simulink model "dsp_channelized_receiver_"  (R2021a)
settings: Solver=VariableStepAuto  StartTime=0.0  StopTime=sim_time  RelTol=1e-3
values from neighbouring files (symbols this model uses):
  sim_time = 1e-3    (= 0.001)    [rx_dsp_core_init_hw.m]
  ts = 1/fs    (= 2.5e-10)    [rx_dsp_core_init_hw.m]
undefined symbols (not defined in the file or in its folder): es1
libraries: xbsIndex_r4 x267, dspsrcs4 x3, simulink x1, dspswit3 x1
(part 1 of 2)
settings Model: ModifiedByFormat=HosseinBehshti  Creator=HosseinBehshti  LastModifiedBy=HosseinBehshti

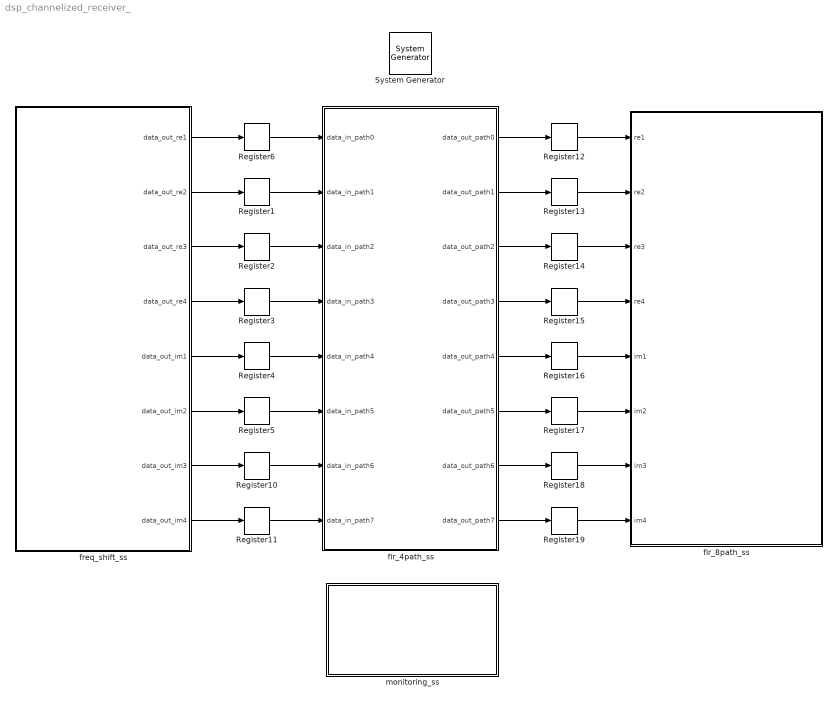
== system dsp_channelized_receiver_ ==
  " System Generator" : xbsIndex_r4/ System Generator  Tag=genX  xilinxfamily=zynquplusRFSOCes1  part=xczu48dr  speed=-2-e-es1  package=fsvg1517  synthesis_tool=Vivado  clock_wrapper=Clock Enables  directory=./netlist  proj_type=Vivado  Synth_file=Vivado Synthesis Defaults  Impl_file=Vivado Implementation Defaults  testbench=off  simulink_period=ts  sysclk_period=2  dcm_input_clock_period=10  incr_netlist=off  trim_vbits=Everywhere in SubSystem  dbl_ovrd=According to Block Masks  core_generation=According to Block Masks  run_coregen=off  deprecated_control=off  eval_field=0  block_type=sysgen
  Register{1..6,10..19} (16 alike) : xbsIndex_r4/Register  init=0  rst=off  en=off  dbl_ovrd=off  block_type=register
  fir_4path_ss : Subsystem
  fir_8path_ss : Subsystem
  freq_shift_ss : Subsystem
  monitoring_ss : Subsystem
  wires:
  Register6/1 -> fir_4path_ss/1(data_in_path0)
  Register1/1 -> fir_4path_ss/2(data_in_path1)
  Register2/1 -> fir_4path_ss/3(data_in_path2)
  Register3/1 -> fir_4path_ss/4(data_in_path3)
  Register4/1 -> fir_4path_ss/5(data_in_path4)
  Register5/1 -> fir_4path_ss/6(data_in_path5)
  Register10/1 -> fir_4path_ss/7(data_in_path6)
  Register11/1 -> fir_4path_ss/8(data_in_path7)
  fir_4path_ss/1(data_out_path0) -> Register12/1
  fir_4path_ss/2(data_out_path1) -> Register13/1
  fir_4path_ss/3(data_out_path2) -> Register14/1
  fir_4path_ss/4(data_out_path3) -> Register15/1
  fir_4path_ss/5(data_out_path4) -> Register16/1
  fir_4path_ss/6(data_out_path5) -> Register17/1
  fir_4path_ss/7(data_out_path6) -> Register18/1
  fir_4path_ss/8(data_out_path7) -> Register19/1
  Register12/1 -> fir_8path_ss/1(re1)
  Register13/1 -> fir_8path_ss/2(re2)
  Register14/1 -> fir_8path_ss/3(re3)
  Register17/1 -> fir_8path_ss/6(im2)
  Register16/1 -> fir_8path_ss/5(im1)
  Register15/1 -> fir_8path_ss/4(re4)
  Register19/1 -> fir_8path_ss/8(im4)
  Register18/1 -> fir_8path_ss/7(im3)
  freq_shift_ss/1(data_out_re1) -> Register6/1
  freq_shift_ss/2(data_out_re2) -> Register1/1
  freq_shift_ss/3(data_out_re3) -> Register2/1
  freq_shift_ss/4(data_out_re4) -> Register3/1
  freq_shift_ss/5(data_out_im1) -> Register4/1
  freq_shift_ss/6(data_out_im2) -> Register5/1
  freq_shift_ss/7(data_out_im3) -> Register10/1
  freq_shift_ss/8(data_out_im4) -> Register11/1

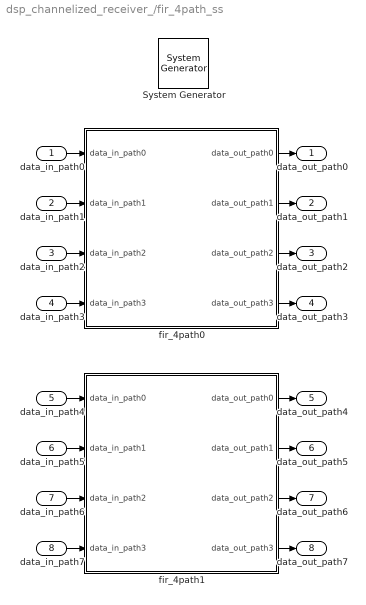
== system dsp_channelized_receiver_/fir_4path_ss ==
  data_in_path0 : Inport
  data_in_path1 : Inport  Port=2
  data_in_path2 : Inport  Port=3
  data_in_path3 : Inport  Port=4
  data_in_path4 : Inport  Port=5
  data_in_path5 : Inport  Port=6
  data_in_path6 : Inport  Port=7
  data_in_path7 : Inport  Port=8
  " System Generator" : xbsIndex_r4/ System Generator  Tag=genX  xilinxfamily=zynquplusRFSOCes1  part=xczu48dr  speed=-2-e-es1  package=fsvg1517  synthesis_tool=Vivado  clock_wrapper=Clock Enables  directory=./netlist  proj_type=Vivado  Synth_file=Vivado Synthesis Defaults  Impl_file=Vivado Implementation Defaults  testbench=off  simulink_period=ts*4  sysclk_period=2*4  dcm_input_clock_period=10  incr_netlist=off  trim_vbits=Everywhere in SubSystem  dbl_ovrd=According to Block Masks  core_generation=According to Block Masks  run_coregen=off  deprecated_control=off  eval_field=0  block_type=sysgen
  fir_4path0 : Subsystem
  fir_4path1 : Subsystem
  data_out_path0 : Outport
  data_out_path1 : Outport  Port=2
  data_out_path2 : Outport  Port=3
  data_out_path3 : Outport  Port=4
  data_out_path4 : Outport  Port=5
  data_out_path5 : Outport  Port=6
  data_out_path6 : Outport  Port=7
  data_out_path7 : Outport  Port=8
  wires:
  data_in_path3/1 -> fir_4path0/4(data_in_path3)
  data_in_path7/1 -> fir_4path1/4(data_in_path3)
  data_in_path4/1 -> fir_4path1/1(data_in_path0)
  fir_4path1/3(data_out_path2) -> data_out_path6/1
  fir_4path1/2(data_out_path1) -> data_out_path5/1
  data_in_path5/1 -> fir_4path1/2(data_in_path1)
  data_in_path6/1 -> fir_4path1/3(data_in_path2)
  fir_4path1/4(data_out_path3) -> data_out_path7/1
  fir_4path1/1(data_out_path0) -> data_out_path4/1
  data_in_path1/1 -> fir_4path0/2(data_in_path1)
  fir_4path0/1(data_out_path0) -> data_out_path0/1
  data_in_path2/1 -> fir_4path0/3(data_in_path2)
  fir_4path0/3(data_out_path2) -> data_out_path2/1
  data_in_path0/1 -> fir_4path0/1(data_in_path0)
  fir_4path0/2(data_out_path1) -> data_out_path1/1
  fir_4path0/4(data_out_path3) -> data_out_path3/1

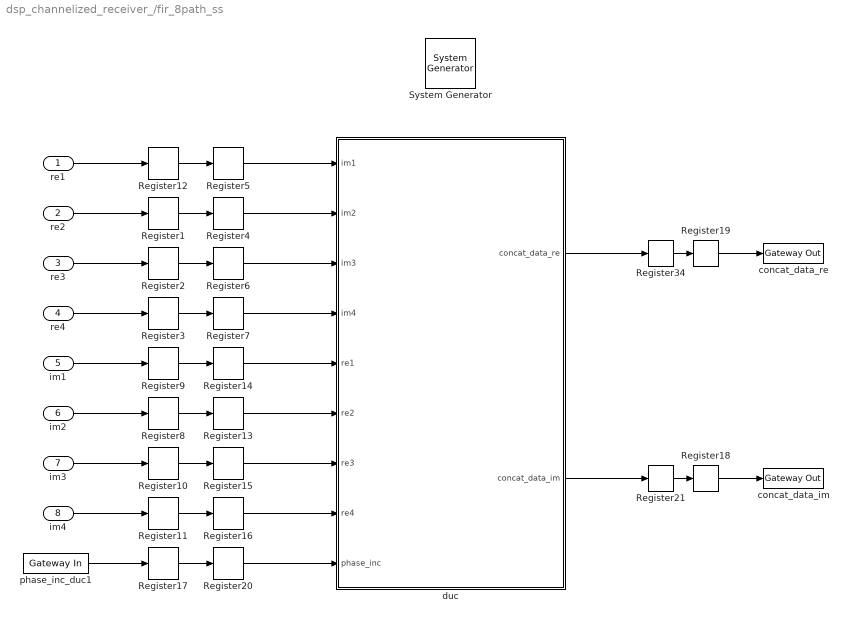
== system dsp_channelized_receiver_/fir_8path_ss ==
  re1 : Inport
  re2 : Inport  Port=2
  re3 : Inport  Port=3
  re4 : Inport  Port=4
  im1 : Inport  Port=5
  im2 : Inport  Port=6
  im3 : Inport  Port=7
  im4 : Inport  Port=8
  " System Generator" : xbsIndex_r4/ System Generator  Tag=genX  xilinxfamily=zynquplusRFSOCes1  part=xczu48dr  speed=-2-e-es1  package=fsvg1517  synthesis_tool=Vivado  clock_wrapper=Clock Enables  directory=./netlist  proj_type=Vivado  Synth_file=Vivado Synthesis Defaults  Impl_file=Vivado Implementation Defaults  testbench=off  simulink_period=ts  sysclk_period=2  dcm_input_clock_period=10  incr_netlist=off  trim_vbits=Everywhere in SubSystem  dbl_ovrd=According to Block Masks  core_generation=According to Block Masks  run_coregen=off  deprecated_control=off  eval_field=0  block_type=sysgen
  Register{1..21,34} (22 alike) : xbsIndex_r4/Register  init=0  rst=off  en=off  dbl_ovrd=off  block_type=register
  concat_data_im : xbsIndex_r4/Gateway Out  inherit_from_input=off  hdl_port=on  rows=1  columns=1  UseAsDAC=off  DACChannel='1'  interface=None  automatic_assignment=on  address_offset=hex2dec('00')  intf_name=''  intf_description=''  timing_constraint=None  locs_specified=off  LOCs={}  io_standard={}  block_type=gatewayout
  concat_data_re : xbsIndex_r4/Gateway Out  inherit_from_input=off  hdl_port=on  rows=1  columns=1  UseAsDAC=off  DACChannel='1'  interface=None  automatic_assignment=on  address_offset=hex2dec('00')  intf_name=''  intf_description=''  timing_constraint=None  locs_specified=off  LOCs={}  io_standard={}  block_type=gatewayout
  duc : Subsystem
  phase_inc_duc1 : xbsIndex_r4/Gateway In  gui_display_data_type=Fixed-point  arith_type=Unsigned  n_bits=ddc_phase_width  bin_pt=ddc_phase_width  preci_type=Single  exp_width=8  frac_width=24  rows=1  columns=1  quantization="Round  (unbiased: +/- Inf)"  overflow=Saturate  period=ts  UseAsADC=off  ADCChannel='1'  interface=None  automatic_assignment=on  address_offset=hex2dec('00')  intf_name=''  intf_description=''  default_value=0  timing_constraint=None  locs_specified=off  LOCs={}  io_standard={}  inherit_from_input=off  hdl_port=on  dbl_ovrd=off  block_type=gatewayin
  wires:
  re1/1 -> Register12/1
  re3/1 -> Register2/1
  re2/1 -> Register1/1
  re4/1 -> Register3/1
  Register12/1 -> Register5/1
  Register1/1 -> Register4/1
  Register2/1 -> Register6/1
  Register3/1 -> Register7/1
  Register11/1 -> Register16/1
  Register10/1 -> Register15/1
  Register8/1 -> Register13/1
  Register9/1 -> Register14/1
  im4/1 -> Register11/1
  im2/1 -> Register8/1
  im3/1 -> Register10/1
  im1/1 -> Register9/1
  Register19/1 -> concat_data_re/1
  Register34/1 -> Register19/1
  Register5/1 -> duc/1(im1)
  Register4/1 -> duc/2(im2)
  Register6/1 -> duc/3(im3)
  Register7/1 -> duc/4(im4)
  Register14/1 -> duc/5(re1)
  Register13/1 -> duc/6(re2)
  Register15/1 -> duc/7(re3)
  Register16/1 -> duc/8(re4)
  duc/1(concat_data_re) -> Register34/1
  Register17/1 -> Register20/1
  Register20/1 -> duc/9(phase_inc)
  phase_inc_duc1/1 -> Register17/1
  Register21/1 -> Register18/1
  Register18/1 -> concat_data_im/1
  duc/2(concat_data_im) -> Register21/1

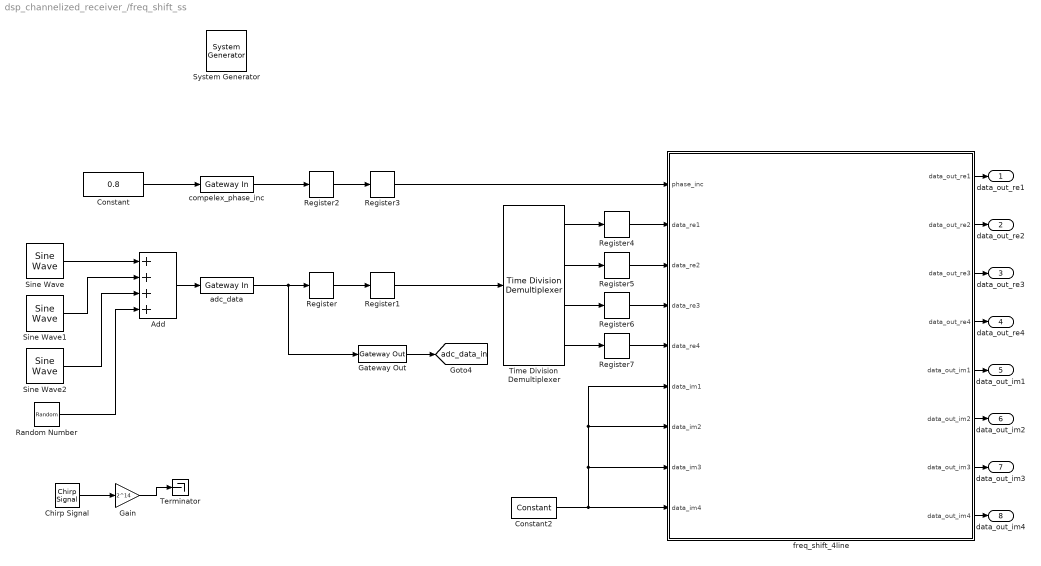
== system dsp_channelized_receiver_/freq_shift_ss ==
  " System Generator" : xbsIndex_r4/ System Generator  Tag=genX  xilinxfamily=zynquplusRFSOCes1  part=xczu48dr  speed=-2-e-es1  package=fsvg1517  synthesis_tool=Vivado  clock_wrapper=Clock Enables  directory=./netlist  proj_type=Vivado  Synth_file=Vivado Synthesis Defaults  Impl_file=Vivado Implementation Defaults  testbench=off  simulink_period=ts  sysclk_period=2  dcm_input_clock_period=10  incr_netlist=off  trim_vbits=Everywhere in SubSystem  dbl_ovrd=According to Block Masks  core_generation=According to Block Masks  run_coregen=off  deprecated_control=off  eval_field=0  block_type=sysgen
  Add : Sum  Inputs=++++
  Chirp Signal : simulink/Sources/Chirp Signal  f1=0.1  T=sim_time  f2=250e6
  Constant : Constant  Value=0.8
  Constant2 : xbsIndex_r4/Constant  const=0  gui_display_data_type=Fixed-point  arith_type=Signed (2's comp)  n_bits=16  bin_pt=0  preci_type=Single  exp_width=8  frac_width=24  explicit_period=on  period=ts*4  equ=P=C  opselect=C  inp2=PCIN>>17  opr=+  inp1=P  carry=CIN  dbl_ovrd=off  block_type=constant
  Gain : Gain  Gain=2^14
  Gateway Out : xbsIndex_r4/Gateway Out  inherit_from_input=off  hdl_port=off  rows=1  columns=1  UseAsDAC=off  DACChannel='1'  interface=None  automatic_assignment=on  address_offset=hex2dec('00')  intf_name=''  intf_description=''  timing_constraint=None  locs_specified=off  LOCs={}  io_standard={}  block_type=gatewayout
  Random Number : RandomNumber  Variance=100  SampleTime=ts
  Register{,1..7} (8 alike) : xbsIndex_r4/Register  init=0  rst=off  en=off  dbl_ovrd=off  block_type=register
  Sine Wave : dspsrcs4/Sine Wave  Amplitude=2^14  Frequency=2.37e9  Phase=0  SampleMode=Discrete  OutComplex=Real  CompMethod=Trigonometric fcn  TableSize=Speed  SampleTime=ts  SamplesPerFrame=1  ResetState=Restart at time zero  OutputFrames=off  dataType=double  wordLen=16  udDataType=sfix(16)  fracBitsMode=Best precision  numFracBits=15  OutDataTypeStr=double  LastOutDataTypeStr=double
  Sine Wave1 : dspsrcs4/Sine Wave  Amplitude=2^13  Frequency=2.4e9  Phase=0  SampleMode=Discrete  OutComplex=Real  CompMethod=Trigonometric fcn  TableSize=Speed  SampleTime=ts  SamplesPerFrame=1  ResetState=Restart at time zero  OutputFrames=off  dataType=double  wordLen=16  udDataType=sfix(16)  fracBitsMode=Best precision  numFracBits=15  OutDataTypeStr=double  LastOutDataTypeStr=double
  Sine Wave2 : dspsrcs4/Sine Wave  Amplitude=2^12  Frequency=2.43e9  Phase=0  SampleMode=Discrete  OutComplex=Real  CompMethod=Trigonometric fcn  TableSize=Speed  SampleTime=ts  SamplesPerFrame=1  ResetState=Restart at time zero  OutputFrames=off  dataType=double  wordLen=16  udDataType=sfix(16)  fracBitsMode=Best precision  numFracBits=15  OutDataTypeStr=double  LastOutDataTypeStr=double
  Terminator : Terminator
  Time Division Demultiplexer : xbsIndex_r4/Time Division Demultiplexer  frame_pattern=[1 1 1 1]  impl_style=Multiple Channel  vin=off  explicit_period=off  dbl_ovrd=off  period=1  block_type=tdd
      settings: infoedit=Samples presented at the input are selected and down-sampled according to the frame sampling pattern specified. The sampled input is presented either as a single or multiple channel at the output.
  adc_data : xbsIndex_r4/Gateway In  gui_display_data_type=Fixed-point  arith_type="Signed  (2's comp)"  n_bits=16  bin_pt=0  preci_type=Single  exp_width=8  frac_width=24  rows=1  columns=1  quantization="Round  (unbiased: +/- Inf)"  overflow=Saturate  period=ts  UseAsADC=off  ADCChannel='1'  interface=None  automatic_assignment=on  address_offset=hex2dec('00')  intf_name=''  intf_description=''  default_value=0  timing_constraint=None  locs_specified=off  LOCs={}  io_standard={}  inherit_from_input=off  hdl_port=on  dbl_ovrd=off  block_type=gatewayin
  compelex_phase_inc : xbsIndex_r4/Gateway In  gui_display_data_type=Fixed-point  arith_type=Unsigned  n_bits=ddc_phase_width  bin_pt=ddc_phase_width  preci_type=Single  exp_width=8  frac_width=24  rows=1  columns=1  quantization="Round  (unbiased: +/- Inf)"  overflow=Saturate  period=ts*4  UseAsADC=off  ADCChannel='1'  interface=None  automatic_assignment=on  address_offset=hex2dec('00')  intf_name=''  intf_description=''  default_value=0  timing_constraint=None  locs_specified=off  LOCs={}  io_standard={}  inherit_from_input=off  hdl_port=on  dbl_ovrd=off  block_type=gatewayin
  freq_shift_4line : Subsystem
  data_out_re1 : Outport
  data_out_re2 : Outport  Port=2
  data_out_re3 : Outport  Port=3
  data_out_re4 : Outport  Port=4
  data_out_im1 : Outport  Port=5
  data_out_im2 : Outport  Port=6
  data_out_im3 : Outport  Port=7
  data_out_im4 : Outport  Port=8
  tag scope: adc_data_in=global
  wires:
  Constant2/1 -> freq_shift_4line/7(data_im2), freq_shift_4line/6(data_im1), freq_shift_4line/8(data_im3), freq_shift_4line/9(data_im4)
  Sine Wave/1 -> Add/1
  Register3/1 -> freq_shift_4line/1(phase_inc)
  Register/1 -> Register1/1
  Gain/1 -> Terminator/1
  Sine Wave2/1 -> Add/3
  Time Division Demultiplexer/1 -> Register4/1
  freq_shift_4line/3(data_out_re3) -> data_out_re3/1
  freq_shift_4line/4(data_out_re4) -> data_out_re4/1
  freq_shift_4line/2(data_out_re2) -> data_out_re2/1
  adc_data/1 -> Gateway Out/1, Register/1
  Time Division Demultiplexer/4 -> Register7/1
  Time Division Demultiplexer/3 -> Register6/1
  Register1/1 -> Time Division Demultiplexer/1
  compelex_phase_inc/1 -> Register2/1
  Register2/1 -> Register3/1
  Gateway Out/1 -> [adc_data_in]
  freq_shift_4line/1(data_out_re1) -> data_out_re1/1
  Chirp Signal/1 -> Gain/1
  Random Number/1 -> Add/4
  Add/1 -> adc_data/1
  Register6/1 -> freq_shift_4line/4(data_re3)
  Constant/1 -> compelex_phase_inc/1
  Sine Wave1/1 -> Add/2
  Register4/1 -> freq_shift_4line/2(data_re1)
  Register7/1 -> freq_shift_4line/5(data_re4)
  freq_shift_4line/8(data_out_im4) -> data_out_im4/1
  Register5/1 -> freq_shift_4line/3(data_re2)
  Time Division Demultiplexer/2 -> Register5/1
  freq_shift_4line/7(data_out_im3) -> data_out_im3/1
  freq_shift_4line/6(data_out_im2) -> data_out_im2/1
  freq_shift_4line/5(data_out_im1) -> data_out_im1/1

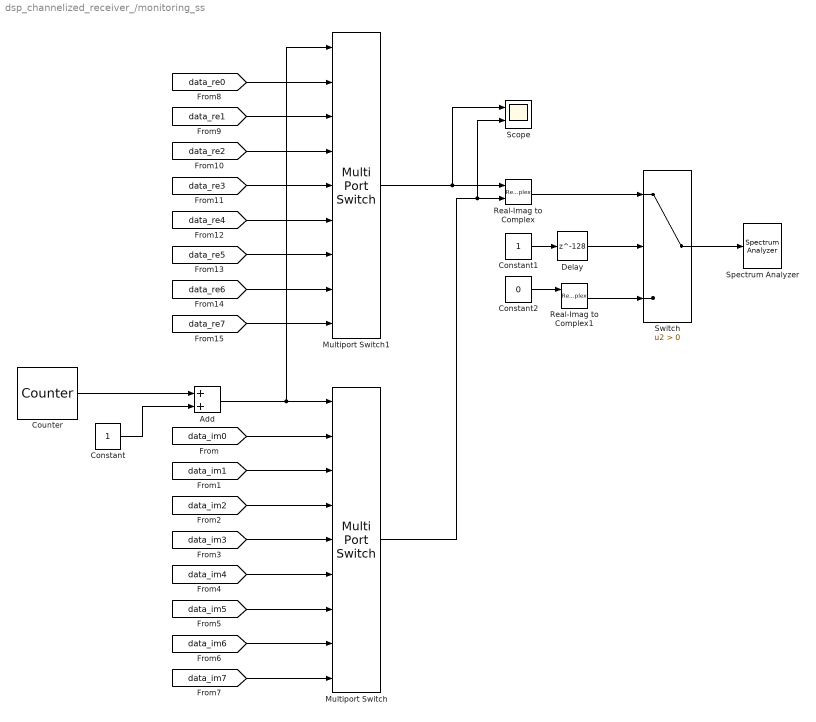
== system dsp_channelized_receiver_/monitoring_ss ==
  Add : Sum
  Constant : Constant
  Constant1 : Constant  SampleTime=ts/8
  Constant2 : Constant  Value=0  SampleTime=ts/8
  Counter : dspswit3/Counter  Direction=Up  CountEvent=Free running  CounterSize=User defined  MaxCount=7  InitialCount=0  Output=Count  HitValue=32  ResetInput=off  SamplesPerFrame=1  Ts=ts*8  CntDtype=double  HitDtype=Logical
  Delay : Delay  DelayLength=128
  Multiport Switch : MultiPortSwitch  Inputs=8
  Multiport Switch1 : MultiPortSwitch  Inputs=8
  Real-Imag to Complex : RealImagToComplex
  Real-Imag to Complex1 : RealImagToComplex
  Scope : Scope  NumInputPorts=2
  Spectrum Analyzer : SpectrumAnalyzer
  Switch : Switch  Criteria=u2 > Threshold
  wires:
  [data_im4] -> Multiport Switch/6
  [data_im3] -> Multiport Switch/5
  Add/1 -> Multiport Switch1/1, Multiport Switch/1
  [data_im0] -> Multiport Switch/2
  Counter/1 -> Add/1
  [data_im1] -> Multiport Switch/3
  [data_im7] -> Multiport Switch/9
  [data_im2] -> Multiport Switch/4
  Constant/1 -> Add/2
  [data_im6] -> Multiport Switch/8
  [data_im5] -> Multiport Switch/7
  [data_re5] -> Multiport Switch1/7
  [data_re6] -> Multiport Switch1/8
  [data_re2] -> Multiport Switch1/4
  [data_re7] -> Multiport Switch1/9
  [data_re1] -> Multiport Switch1/3
  [data_re3] -> Multiport Switch1/5
  [data_re4] -> Multiport Switch1/6
  [data_re0] -> Multiport Switch1/2
  Multiport Switch1/1 -> Scope/1, Real-Imag to Complex/1
  Multiport Switch/1 -> Scope/2, Real-Imag to Complex/2
  Switch/1 -> Spectrum Analyzer/1
  Real-Imag to Complex/1 -> Switch/1
  Constant1/1 -> Delay/1
  Delay/1 -> Switch/2
  Constant2/1 -> Real-Imag to Complex1/1
  Real-Imag to Complex1/1 -> Switch/3

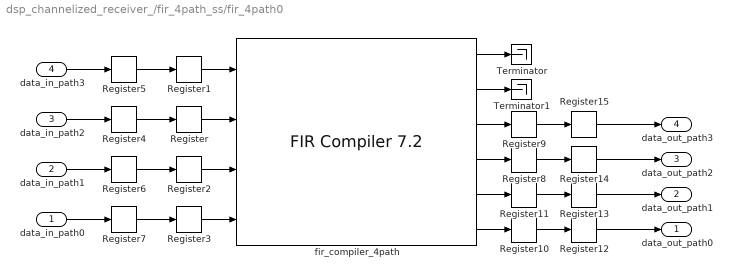
== system dsp_channelized_receiver_/fir_4path_ss/fir_4path0 ==
  data_in_path0 : Inport
  data_in_path1 : Inport  Port=2
  data_in_path2 : Inport  Port=3
  data_in_path3 : Inport  Port=4
  Register{,1..15} (16 alike) : xbsIndex_r4/Register  init=0  rst=off  en=off  dbl_ovrd=off  block_type=register
  Terminator : Terminator
  Terminator1 : Terminator
  fir_compiler_4path : xbsIndex_r4/FIR Compiler 7.2   coefficientvector=lpf1_coefficient  coefficient_sets=1  coefficient_reload=off  filter_type=Single_Rate  rate_change_type=Integer  interpolation_rate=1  decimation_rate=1  zero_pack_factor=1  channel_sequence=Basic  number_channels=1  pattern_list='P4-0,P4-1,P4-2,P4-3,P4-4'  number_paths=4  ratespecification=Maximum_Possible  sampleperiod=4  hardwareoversamplingrate=1  coefficient_sign=Signed  quantization=Quantize_Only  coefficient_width=16  bestprecision=on  coefficient_fractional_bits=18  coefficient_structure=Inferred  output_rounding_mode=Truncate_LSBs  output_width=16  filter_architecture=Systolic_Multiply_Accumulate  optimization_goal=Speed  optimization_list='Data_Path_Fanout,Pre-Adder_Pipeline,Coefficient_Fanout,Control_Path_Fanout,Control_Column_Fanout,Control_Broadcast_Fanout,Control_LUT_Pipeline,No_BRAM_Read_First_Mode,Optimal_Column_Lengths,Other'  data_buffer_type=Automatic  coefficient_buffer_type=Automatic  input_buffer_type=Automatic  output_buffer_type=Automatic  preference_for_other_storage=Automatic  multi_column_support=Automatic  columnconfig='32'  inter_column_pipe_length=4  data_has_tlast=Not_Required  m_data_has_tready=off  s_data_has_fifo=off  s_data_has_tuser=Not_Required  m_data_has_tuser=Not_Required  s_config_sync_mode=On_Vector  s_config_method=Single  num_reload_slots=1  has_aclken=off  has_aresetn=off  infoeditControl=ARESETn must be asserted for a minimum of 2 cycles  reset_data_vector=on  trim_axipin_name=on  simulation_type=hybrid_sim  simulation_model=sysgen:xfirv7_2_cmodel  data_path_portlist={ 's_axis_data_tdata', 'm_axis_data_tdata' }  passband_min=0.0  passband_max=0.5  stopband_min=0.5  stopband_max=1.0  filter_selection=1  gui_behaviour='Sysgen_GUI'  data_sign=Signed  data_width=16  data_fractional_bits=0  data_tuser_width=1  wrapper_available=true  ip_wrap_arbitrary_binary_point=true  ip_name=FIR Compiler  ip_version=7.2  dsptool_ready=true  ipcore_usecache=true  ipcore_useipmodelcache=true  port_translation_map={ 'aclken' => 'en', 'aresetn' => 'rst' }  run_core_at_system_period=true  ipcore_xco_need_fpga_part=true  block_type=fir_compiler_v7_2
      settings: infoedit=Maximum Possible : Maximizes oversampling rate. Abstracted input handshake (no s_data_tvalid) and automatic rate propagation.<br>Hardware Oversampling Rate : Specifies oversampling rate relative to the input sample period. Abstracted input handshake (no s_data_tvalid) and automatic rate propagation.<br>Input/Output Sample Period : Specifies absolute oversampling rate. No input handshake abstraction (exposes s_data_tvalid) and no rate propagation.
  data_out_path0 : Outport
  data_out_path1 : Outport  Port=2
  data_out_path2 : Outport  Port=3
  data_out_path3 : Outport  Port=4
  wires:
  Register3/1 -> fir_compiler_4path/4
  Register11/1 -> Register13/1
  Register/1 -> fir_compiler_4path/2
  Register7/1 -> Register3/1
  Register9/1 -> Register15/1
  fir_compiler_4path/4 -> Register8/1
  Register6/1 -> Register2/1
  Register5/1 -> Register1/1
  Register2/1 -> fir_compiler_4path/3
  Register10/1 -> Register12/1
  data_in_path1/1 -> Register6/1
  fir_compiler_4path/5 -> Register11/1
  Register12/1 -> data_out_path0/1
  fir_compiler_4path/1 -> Terminator/1
  fir_compiler_4path/2 -> Terminator1/1
  Register4/1 -> Register/1
  Register8/1 -> Register14/1
  Register1/1 -> fir_compiler_4path/1
  data_in_path3/1 -> Register5/1
  fir_compiler_4path/3 -> Register9/1
  fir_compiler_4path/6 -> Register10/1
  data_in_path0/1 -> Register7/1
  Register13/1 -> data_out_path1/1
  Register14/1 -> data_out_path2/1
  Register15/1 -> data_out_path3/1
  data_in_path2/1 -> Register4/1

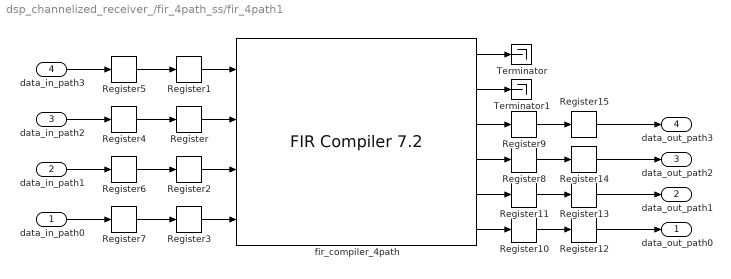
== system dsp_channelized_receiver_/fir_4path_ss/fir_4path1 ==
  data_in_path0 : Inport
  data_in_path1 : Inport  Port=2
  data_in_path2 : Inport  Port=3
  data_in_path3 : Inport  Port=4
  Register{,1..15} (16 alike) : xbsIndex_r4/Register  init=0  rst=off  en=off  dbl_ovrd=off  block_type=register
  Terminator : Terminator
  Terminator1 : Terminator
  fir_compiler_4path : xbsIndex_r4/FIR Compiler 7.2   coefficientvector=lpf1_coefficient  coefficient_sets=1  coefficient_reload=off  filter_type=Single_Rate  rate_change_type=Integer  interpolation_rate=1  decimation_rate=1  zero_pack_factor=1  channel_sequence=Basic  number_channels=1  pattern_list='P4-0,P4-1,P4-2,P4-3,P4-4'  number_paths=4  ratespecification=Maximum_Possible  sampleperiod=4  hardwareoversamplingrate=1  coefficient_sign=Signed  quantization=Quantize_Only  coefficient_width=16  bestprecision=on  coefficient_fractional_bits=18  coefficient_structure=Inferred  output_rounding_mode=Truncate_LSBs  output_width=16  filter_architecture=Systolic_Multiply_Accumulate  optimization_goal=Speed  optimization_list='Data_Path_Fanout,Pre-Adder_Pipeline,Coefficient_Fanout,Control_Path_Fanout,Control_Column_Fanout,Control_Broadcast_Fanout,Control_LUT_Pipeline,No_BRAM_Read_First_Mode,Optimal_Column_Lengths,Other'  data_buffer_type=Automatic  coefficient_buffer_type=Automatic  input_buffer_type=Automatic  output_buffer_type=Automatic  preference_for_other_storage=Automatic  multi_column_support=Automatic  columnconfig='32'  inter_column_pipe_length=4  data_has_tlast=Not_Required  m_data_has_tready=off  s_data_has_fifo=off  s_data_has_tuser=Not_Required  m_data_has_tuser=Not_Required  s_config_sync_mode=On_Vector  s_config_method=Single  num_reload_slots=1  has_aclken=off  has_aresetn=off  infoeditControl=ARESETn must be asserted for a minimum of 2 cycles  reset_data_vector=on  trim_axipin_name=on  simulation_type=hybrid_sim  simulation_model=sysgen:xfirv7_2_cmodel  data_path_portlist={ 's_axis_data_tdata', 'm_axis_data_tdata' }  passband_min=0.0  passband_max=0.5  stopband_min=0.5  stopband_max=1.0  filter_selection=1  gui_behaviour='Sysgen_GUI'  data_sign=Signed  data_width=16  data_fractional_bits=0  data_tuser_width=1  wrapper_available=true  ip_wrap_arbitrary_binary_point=true  ip_name=FIR Compiler  ip_version=7.2  dsptool_ready=true  ipcore_usecache=true  ipcore_useipmodelcache=true  port_translation_map={ 'aclken' => 'en', 'aresetn' => 'rst' }  run_core_at_system_period=true  ipcore_xco_need_fpga_part=true  block_type=fir_compiler_v7_2
      settings: infoedit=Maximum Possible : Maximizes oversampling rate. Abstracted input handshake (no s_data_tvalid) and automatic rate propagation.<br>Hardware Oversampling Rate : Specifies oversampling rate relative to the input sample period. Abstracted input handshake (no s_data_tvalid) and automatic rate propagation.<br>Input/Output Sample Period : Specifies absolute oversampling rate. No input handshake abstraction (exposes s_data_tvalid) and no rate propagation.
  data_out_path0 : Outport
  data_out_path1 : Outport  Port=2
  data_out_path2 : Outport  Port=3
  data_out_path3 : Outport  Port=4
  wires:
  data_in_path2/1 -> Register4/1
  Register15/1 -> data_out_path3/1
  Register14/1 -> data_out_path2/1
  Register13/1 -> data_out_path1/1
  data_in_path0/1 -> Register7/1
  fir_compiler_4path/6 -> Register10/1
  fir_compiler_4path/3 -> Register9/1
  data_in_path3/1 -> Register5/1
  Register1/1 -> fir_compiler_4path/1
  Register8/1 -> Register14/1
  Register4/1 -> Register/1
  fir_compiler_4path/2 -> Terminator1/1
  fir_compiler_4path/1 -> Terminator/1
  Register12/1 -> data_out_path0/1
  fir_compiler_4path/5 -> Register11/1
  data_in_path1/1 -> Register6/1
  Register10/1 -> Register12/1
  Register2/1 -> fir_compiler_4path/3
  Register5/1 -> Register1/1
  Register6/1 -> Register2/1
  fir_compiler_4path/4 -> Register8/1
  Register9/1 -> Register15/1
  Register7/1 -> Register3/1
  Register/1 -> fir_compiler_4path/2
  Register11/1 -> Register13/1
  Register3/1 -> fir_compiler_4path/4

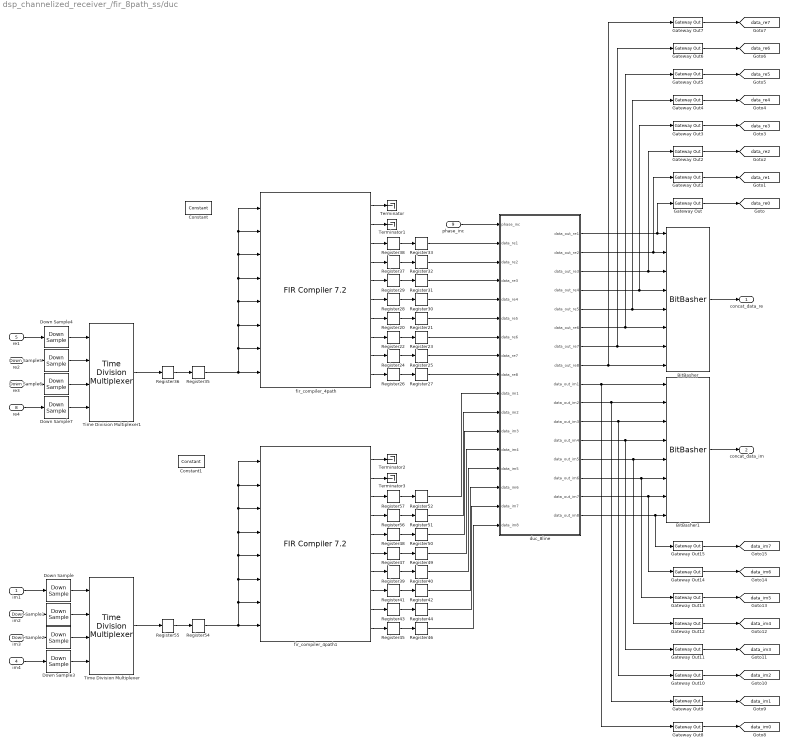
== system dsp_channelized_receiver_/fir_8path_ss/duc ==
  im1 : Inport
  im2 : Inport  Port=2
  im3 : Inport  Port=3
  im4 : Inport  Port=4
  re1 : Inport  Port=5
  re2 : Inport  Port=6
  re3 : Inport  Port=7
  re4 : Inport  Port=8
  phase_inc : Inport  Port=9
  BitBasher : xbsIndex_r4/BitBasher  bitexpr=out={in0,in1,in2,in3,in4,in5,in6,in7}  display_expr=off  sr_1=out  arith_type1=Unsigned  bin_pt1=0  sr_2=2  arith_type2=Unsigned  bin_pt2=0  sr_3=3  arith_type3=Unsigned  bin_pt3=0  sr_4=4  arith_type4=Unsigned  bin_pt4=0  dbl_ovrd=off  block_type=bitbasher
  BitBasher1 : xbsIndex_r4/BitBasher  bitexpr=out={in0,in1,in2,in3,in4,in5,in6,in7}  display_expr=off  sr_1=out  arith_type1=Unsigned  bin_pt1=0  sr_2=2  arith_type2=Unsigned  bin_pt2=0  sr_3=3  arith_type3=Unsigned  bin_pt3=0  sr_4=4  arith_type4=Unsigned  bin_pt4=0  dbl_ovrd=off  block_type=bitbasher
  Constant : xbsIndex_r4/Constant  const=0  gui_display_data_type=Fixed-point  arith_type=Signed (2's comp)  n_bits=16  bin_pt=0  preci_type=Single  exp_width=8  frac_width=24  explicit_period=on  period=ts  equ=P=C  opselect=C  inp2=PCIN>>17  opr=+  inp1=P  carry=CIN  dbl_ovrd=off  block_type=constant
  Constant1 : xbsIndex_r4/Constant  const=0  gui_display_data_type=Fixed-point  arith_type=Signed (2's comp)  n_bits=16  bin_pt=0  preci_type=Single  exp_width=8  frac_width=24  explicit_period=on  period=ts  equ=P=C  opselect=C  inp2=PCIN>>17  opr=+  inp1=P  carry=CIN  dbl_ovrd=off  block_type=constant
  Down Sample{,1..7} (8 alike) : xbsIndex_r4/Down Sample  sample_ratio=4  sample_phase="Last Value of Frame  (most efficient)"  en=off  rst=off  latency=1  dbl_ovrd=off  block_type=dsamp
  Gateway Out{,1..15} (16 alike) : xbsIndex_r4/Gateway Out  inherit_from_input=off  hdl_port=off  rows=1  columns=1  UseAsDAC=off  DACChannel='1'  interface=None  automatic_assignment=on  address_offset=hex2dec('00')  intf_name=''  intf_description=''  timing_constraint=None  locs_specified=off  LOCs={}  io_standard={}  block_type=gatewayout
  Register{20..33,35..52,54..57} (36 alike) : xbsIndex_r4/Register  init=0  rst=off  en=off  dbl_ovrd=off  block_type=register
  Terminator{,1..3} (4 alike) : Terminator
  Time Division Multiplexer : xbsIndex_r4/Time Division Multiplexer  inputs=4  vin=off  Optimization=Resource  explicit_period=off  period=1  dbl_ovrd=off  block_type=tdm
      settings: infoedit="Multiple inputs are sampled and  presented serially at the output."
  Time Division Multiplexer1 : xbsIndex_r4/Time Division Multiplexer  inputs=4  vin=off  Optimization=Resource  explicit_period=off  period=1  dbl_ovrd=off  block_type=tdm
      settings: infoedit="Multiple inputs are sampled and  presented serially at the output."
  duc_8line : Subsystem
  fir_compiler_4path : xbsIndex_r4/FIR Compiler 7.2   coefficientvector=lpf2_coefficient  coefficient_sets=1  coefficient_reload=off  filter_type=Single_Rate  rate_change_type=Integer  interpolation_rate=1  decimation_rate=1  zero_pack_factor=1  channel_sequence=Basic  number_channels=1  pattern_list='P4-0,P4-1,P4-2,P4-3,P4-4'  number_paths=8  ratespecification=Maximum_Possible  sampleperiod=1  hardwareoversamplingrate=1  coefficient_sign=Signed  quantization=Quantize_Only  coefficient_width=16  bestprecision=on  coefficient_fractional_bits=18  coefficient_structure=Inferred  output_rounding_mode=Truncate_LSBs  output_width=16  filter_architecture=Systolic_Multiply_Accumulate  optimization_goal=Speed  optimization_list='Data_Path_Fanout,Pre-Adder_Pipeline,Coefficient_Fanout,Control_Path_Fanout,Control_Column_Fanout,Control_Broadcast_Fanout,Control_LUT_Pipeline,No_BRAM_Read_First_Mode,Optimal_Column_Lengths,Other'  data_buffer_type=Automatic  coefficient_buffer_type=Automatic  input_buffer_type=Automatic  output_buffer_type=Automatic  preference_for_other_storage=Automatic  multi_column_support=Automatic  columnconfig='64'  inter_column_pipe_length=4  data_has_tlast=Not_Required  m_data_has_tready=off  s_data_has_fifo=off  s_data_has_tuser=Not_Required  m_data_has_tuser=Not_Required  s_config_sync_mode=On_Vector  s_config_method=Single  num_reload_slots=1  has_aclken=off  has_aresetn=off  infoeditControl=ARESETn must be asserted for a minimum of 2 cycles  reset_data_vector=on  trim_axipin_name=on  simulation_type=hybrid_sim  simulation_model=sysgen:xfirv7_2_cmodel  data_path_portlist={ 's_axis_data_tdata', 'm_axis_data_tdata' }  passband_min=0.0  passband_max=0.5  stopband_min=0.5  stopband_max=1.0  filter_selection=1  gui_behaviour='Sysgen_GUI'  data_sign=Signed  data_width=16  data_fractional_bits=0  data_tuser_width=1  wrapper_available=true  ip_wrap_arbitrary_binary_point=true  ip_name=FIR Compiler  ip_version=7.2  dsptool_ready=true  ipcore_usecache=true  ipcore_useipmodelcache=true  port_translation_map={ 'aclken' => 'en', 'aresetn' => 'rst' }  run_core_at_system_period=true  ipcore_xco_need_fpga_part=true  block_type=fir_compiler_v7_2
      settings: infoedit=Maximum Possible : Maximizes oversampling rate. Abstracted input handshake (no s_data_tvalid) and automatic rate propagation.<br>Hardware Oversampling Rate : Specifies oversampling rate relative to the input sample period. Abstracted input handshake (no s_data_tvalid) and automatic rate propagation.<br>Input/Output Sample Period : Specifies absolute oversampling rate. No input handshake abstraction (exposes s_data_tvalid) and no rate propagation.
  fir_compiler_4path1 : xbsIndex_r4/FIR Compiler 7.2   coefficientvector=lpf2_coefficient  coefficient_sets=1  coefficient_reload=off  filter_type=Single_Rate  rate_change_type=Integer  interpolation_rate=1  decimation_rate=1  zero_pack_factor=1  channel_sequence=Basic  number_channels=1  pattern_list='P4-0,P4-1,P4-2,P4-3,P4-4'  number_paths=8  ratespecification=Maximum_Possible  sampleperiod=1  hardwareoversamplingrate=1  coefficient_sign=Signed  quantization=Quantize_Only  coefficient_width=16  bestprecision=on  coefficient_fractional_bits=18  coefficient_structure=Inferred  output_rounding_mode=Truncate_LSBs  output_width=16  filter_architecture=Systolic_Multiply_Accumulate  optimization_goal=Speed  optimization_list='Data_Path_Fanout,Pre-Adder_Pipeline,Coefficient_Fanout,Control_Path_Fanout,Control_Column_Fanout,Control_Broadcast_Fanout,Control_LUT_Pipeline,No_BRAM_Read_First_Mode,Optimal_Column_Lengths,Other'  data_buffer_type=Automatic  coefficient_buffer_type=Automatic  input_buffer_type=Automatic  output_buffer_type=Automatic  preference_for_other_storage=Automatic  multi_column_support=Automatic  columnconfig='64'  inter_column_pipe_length=4  data_has_tlast=Not_Required  m_data_has_tready=off  s_data_has_fifo=off  s_data_has_tuser=Not_Required  m_data_has_tuser=Not_Required  s_config_sync_mode=On_Vector  s_config_method=Single  num_reload_slots=1  has_aclken=off  has_aresetn=off  infoeditControl=ARESETn must be asserted for a minimum of 2 cycles  reset_data_vector=on  trim_axipin_name=on  simulation_type=hybrid_sim  simulation_model=sysgen:xfirv7_2_cmodel  data_path_portlist={ 's_axis_data_tdata', 'm_axis_data_tdata' }  passband_min=0.0  passband_max=0.5  stopband_min=0.5  stopband_max=1.0  filter_selection=1  gui_behaviour='Sysgen_GUI'  data_sign=Signed  data_width=16  data_fractional_bits=0  data_tuser_width=1  wrapper_available=true  ip_wrap_arbitrary_binary_point=true  ip_name=FIR Compiler  ip_version=7.2  dsptool_ready=true  ipcore_usecache=true  ipcore_useipmodelcache=true  port_translation_map={ 'aclken' => 'en', 'aresetn' => 'rst' }  run_core_at_system_period=true  ipcore_xco_need_fpga_part=true  block_type=fir_compiler_v7_2
      settings: infoedit=Maximum Possible : Maximizes oversampling rate. Abstracted input handshake (no s_data_tvalid) and automatic rate propagation.<br>Hardware Oversampling Rate : Specifies oversampling rate relative to the input sample period. Abstracted input handshake (no s_data_tvalid) and automatic rate propagation.<br>Input/Output Sample Period : Specifies absolute oversampling rate. No input handshake abstraction (exposes s_data_tvalid) and no rate propagation.
  concat_data_re : Outport
  concat_data_im : Outport  Port=2
  tag scope: data_im0=global, data_im1=global, data_im2=global, data_im3=global, data_im4=global, data_im5=global, data_im6=global, data_im7=global, data_re0=global, data_re1=global, data_re2=global, data_re3=global, data_re4=global, data_re5=global, data_re6=global, data_re7=global
  wires:
  fir_compiler_4path1/3 -> Register57/1
  Register56/1 -> Register51/1
  Register35/1 -> fir_compiler_4path/1, fir_compiler_4path/2, fir_compiler_4path/3, fir_compiler_4path/4, fir_compiler_4path/5, fir_compiler_4path/6, fir_compiler_4path/7, fir_compiler_4path/8
  Register57/1 -> Register52/1
  Register41/1 -> Register42/1
  Register54/1 -> fir_compiler_4path1/1, fir_compiler_4path1/2, fir_compiler_4path1/3, fir_compiler_4path1/4, fir_compiler_4path1/5, fir_compiler_4path1/6, fir_compiler_4path1/7, fir_compiler_4path1/8
  fir_compiler_4path/3 -> Register38/1
  BitBasher/1 -> concat_data_re/1
  Register24/1 -> Register25/1
  fir_compiler_4path/1 -> Terminator/1
  fir_compiler_4path1/2 -> Terminator3/1
  Register36/1 -> Register35/1
  re3/1 -> Down Sample6/1
  Register45/1 -> Register46/1
  fir_compiler_4path/4 -> Register37/1
  Time Division Multiplexer/1 -> Register55/1
  fir_compiler_4path/9 -> Register24/1
  re1/1 -> Down Sample4/1
  Time Division Multiplexer1/1 -> Register36/1
  fir_compiler_4path/7 -> Register20/1
  Register28/1 -> Register30/1
  Register26/1 -> Register27/1
  Register39/1 -> Register40/1
  fir_compiler_4path1/10 -> Register45/1
  fir_compiler_4path/6 -> Register28/1
  fir_compiler_4path1/5 -> Register48/1
  im2/1 -> Down Sample1/1
  Register43/1 -> Register44/1
  Down Sample3/1 -> Time Division Multiplexer/4
  fir_compiler_4path1/1 -> Terminator2/1
  Down Sample4/1 -> Time Division Multiplexer1/1
  im1/1 -> Down Sample/1
  Register29/1 -> Register31/1
  Register47/1 -> Register49/1
  fir_compiler_4path/8 -> Register22/1
  Down Sample5/1 -> Time Division Multiplexer1/2
  Register37/1 -> Register32/1
  fir_compiler_4path/10 -> Register26/1
  fir_compiler_4path1/6 -> Register47/1
  Register20/1 -> Register21/1
  fir_compiler_4path1/4 -> Register56/1
  Register48/1 -> Register50/1
  fir_compiler_4path1/8 -> Register41/1
  fir_compiler_4path/5 -> Register29/1
  Register38/1 -> Register33/1
  Register22/1 -> Register23/1
  fir_compiler_4path/2 -> Terminator1/1
  fir_compiler_4path1/9 -> Register43/1
  fir_compiler_4path1/7 -> Register39/1
  Register55/1 -> Register54/1
  Down Sample7/1 -> Time Division Multiplexer1/4
  Down Sample6/1 -> Time Division Multiplexer1/3
  Down Sample2/1 -> Time Division Multiplexer/3
  Down Sample1/1 -> Time Division Multiplexer/2
  Down Sample/1 -> Time Division Multiplexer/1
  im3/1 -> Down Sample2/1
  im4/1 -> Down Sample3/1
  re4/1 -> Down Sample7/1
  re2/1 -> Down Sample5/1
  Register33/1 -> duc_8line/2(data_re1)
  Register32/1 -> duc_8line/3(data_re2)
  Register31/1 -> duc_8line/4(data_re3)
  Register30/1 -> duc_8line/5(data_re4)
  Register21/1 -> duc_8line/6(data_re5)
  Register23/1 -> duc_8line/7(data_re6)
  Register25/1 -> duc_8line/8(data_re7)
  Register27/1 -> duc_8line/9(data_re8)
  Register52/1 -> duc_8line/10(data_im1)
  Register51/1 -> duc_8line/11(data_im2)
  Register50/1 -> duc_8line/12(data_im3)
  Register49/1 -> duc_8line/13(data_im4)
  Register40/1 -> duc_8line/14(data_im5)
  Register42/1 -> duc_8line/15(data_im6)
  Register44/1 -> duc_8line/16(data_im7)
  Register46/1 -> duc_8line/17(data_im8)
  duc_8line/1(data_out_re1) -> Gateway Out/1, BitBasher/1
  duc_8line/2(data_out_re2) -> Gateway Out1/1, BitBasher/2
  duc_8line/3(data_out_re3) -> Gateway Out2/1, BitBasher/3
  duc_8line/4(data_out_re4) -> Gateway Out3/1, BitBasher/4
  duc_8line/5(data_out_re5) -> Gateway Out4/1, BitBasher/5
  duc_8line/6(data_out_re6) -> Gateway Out5/1, BitBasher/6
  duc_8line/7(data_out_re7) -> Gateway Out6/1, BitBasher/7
  duc_8line/8(data_out_re8) -> Gateway Out7/1, BitBasher/8
  duc_8line/9(data_out_im1) -> Gateway Out8/1, BitBasher1/1
  duc_8line/10(data_out_im2) -> Gateway Out9/1, BitBasher1/2
  duc_8line/11(data_out_im3) -> Gateway Out10/1, BitBasher1/3
  duc_8line/12(data_out_im4) -> Gateway Out11/1, BitBasher1/4
  duc_8line/13(data_out_im5) -> Gateway Out12/1, BitBasher1/5
  duc_8line/14(data_out_im6) -> Gateway Out13/1, BitBasher1/6
  duc_8line/15(data_out_im7) -> Gateway Out14/1, BitBasher1/7
  duc_8line/16(data_out_im8) -> Gateway Out15/1, BitBasher1/8
  BitBasher1/1 -> concat_data_im/1
  phase_inc/1 -> duc_8line/1(phase_inc)
  Gateway Out/1 -> [data_re0]
  Gateway Out1/1 -> [data_re1]
  Gateway Out3/1 -> [data_re3]
  Gateway Out2/1 -> [data_re2]
  Gateway Out7/1 -> [data_re7]
  Gateway Out6/1 -> [data_re6]
  Gateway Out5/1 -> [data_re5]
  Gateway Out4/1 -> [data_re4]
  Gateway Out14/1 -> [data_im6]
  Gateway Out10/1 -> [data_im2]
  Gateway Out13/1 -> [data_im5]
  Gateway Out8/1 -> [data_im0]
  Gateway Out9/1 -> [data_im1]
  Gateway Out15/1 -> [data_im7]
  Gateway Out12/1 -> [data_im4]
  Gateway Out11/1 -> [data_im3]

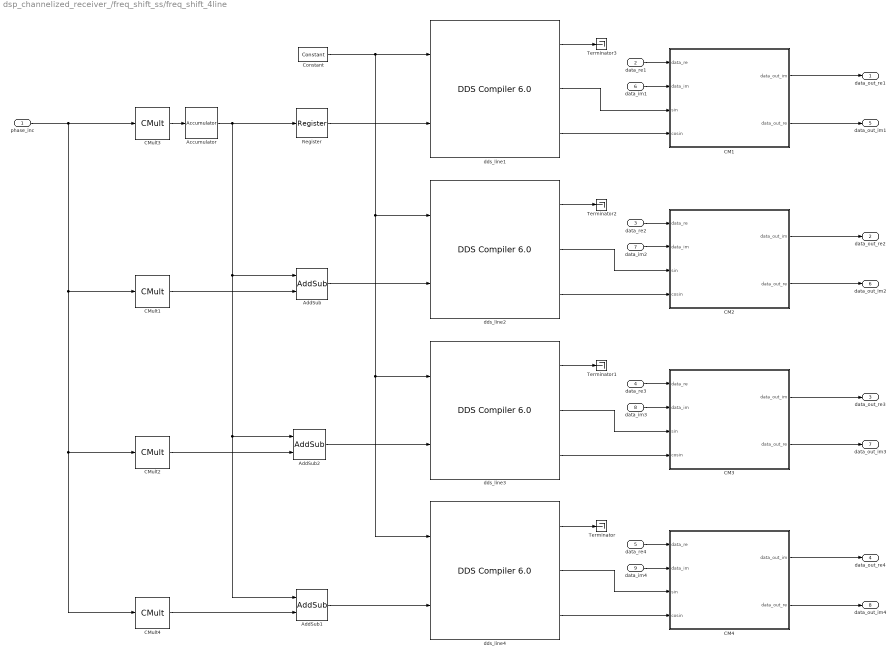
== system dsp_channelized_receiver_/freq_shift_ss/freq_shift_4line ==
  phase_inc : Inport
  data_re1 : Inport  Port=2
  data_re2 : Inport  Port=3
  data_re3 : Inport  Port=4
  data_re4 : Inport  Port=5
  data_im1 : Inport  Port=6
  data_im2 : Inport  Port=7
  data_im3 : Inport  Port=8
  data_im4 : Inport  Port=9
  Accumulator : xbsIndex_r4/Accumulator  operation=Add  n_bits=ddc_phase_width  overflow=Wrap  scale=1  rst=off  hasbypass=off  infoeditControl=reset for floating point data type must be asserted for a minimum of 2 cycles  en=off  latency=1  msb_inp=100  msb=100  lsb=-100  use_behavioral_HDL=on  implementation=Fabric  dbl_ovrd=off  block_type=accum
  AddSub : xbsIndex_r4/AddSub  mode=Addition  use_carryin=off  use_carryout=off  en=off  latency=1  precision=User Defined  arith_type=Unsigned  n_bits=ddc_phase_width  bin_pt=ddc_phase_width  quantization="Round  (unbiased: +/- Inf)"  overflow=Wrap  use_behavioral_HDL=off  hw_selection=Fabric  pipelined=off  dbl_ovrd=off  block_type=addsub
  AddSub1 : xbsIndex_r4/AddSub  mode=Addition  use_carryin=off  use_carryout=off  en=off  latency=1  precision=User Defined  arith_type=Unsigned  n_bits=ddc_phase_width  bin_pt=ddc_phase_width  quantization="Round  (unbiased: +/- Inf)"  overflow=Wrap  use_behavioral_HDL=off  hw_selection=Fabric  pipelined=off  dbl_ovrd=off  block_type=addsub
  AddSub2 : xbsIndex_r4/AddSub  mode=Addition  use_carryin=off  use_carryout=off  en=off  latency=1  precision=User Defined  arith_type=Unsigned  n_bits=ddc_phase_width  bin_pt=ddc_phase_width  quantization="Round  (unbiased: +/- Inf)"  overflow=Wrap  use_behavioral_HDL=off  hw_selection=Fabric  pipelined=off  dbl_ovrd=off  block_type=addsub
  CM1 : Subsystem
  CM2 : Subsystem
  CM3 : Subsystem
  CM4 : Subsystem
  CMult1 : xbsIndex_r4/CMult  const=1  gui_display_data_type=Fixed-point  const_n_bits=4  const_bin_pt=0  float_type=Single  exp_bits=8  fraction_bits=24  en=off  latency=1  precision=User Defined  arith_type=Unsigned  n_bits=ddc_phase_width  bin_pt=ddc_phase_width  quantization="Round  (unbiased: +/- Inf)"  overflow=Wrap  use_behavioral_HDL=off  mem_type=Distributed RAM  pipeline=off  dbl_ovrd=off  block_type=cmult
  CMult2 : xbsIndex_r4/CMult  const=2  gui_display_data_type=Fixed-point  const_n_bits=4  const_bin_pt=0  float_type=Single  exp_bits=8  fraction_bits=24  en=off  latency=1  precision=User Defined  arith_type=Unsigned  n_bits=ddc_phase_width  bin_pt=ddc_phase_width  quantization="Round  (unbiased: +/- Inf)"  overflow=Wrap  use_behavioral_HDL=off  mem_type=Distributed RAM  pipeline=off  dbl_ovrd=off  block_type=cmult
  CMult3 : xbsIndex_r4/CMult  const=4  gui_display_data_type=Fixed-point  const_n_bits=4  const_bin_pt=0  float_type=Single  exp_bits=8  fraction_bits=24  en=off  latency=1  precision=User Defined  arith_type=Unsigned  n_bits=ddc_phase_width  bin_pt=ddc_phase_width  quantization="Round  (unbiased: +/- Inf)"  overflow=Wrap  use_behavioral_HDL=off  mem_type=Distributed RAM  pipeline=off  dbl_ovrd=off  block_type=cmult
  CMult4 : xbsIndex_r4/CMult  const=3  gui_display_data_type=Fixed-point  const_n_bits=4  const_bin_pt=0  float_type=Single  exp_bits=8  fraction_bits=24  en=off  latency=1  precision=User Defined  arith_type=Unsigned  n_bits=ddc_phase_width  bin_pt=ddc_phase_width  quantization="Round  (unbiased: +/- Inf)"  overflow=Wrap  use_behavioral_HDL=off  mem_type=Distributed RAM  pipeline=off  dbl_ovrd=off  block_type=cmult
  Constant : xbsIndex_r4/Constant  const=1  gui_display_data_type=Boolean  arith_type=Boolean  n_bits=16  bin_pt=14  preci_type=Single  exp_width=8  frac_width=24  explicit_period=on  period=ts*4  equ=P=C  opselect=C  inp2=PCIN>>17  opr=+  inp1=P  carry=CIN  dbl_ovrd=off  block_type=constant
  Register : xbsIndex_r4/Register  init=0  rst=off  en=off  dbl_ovrd=off  block_type=register
  Terminator{,1..3} (4 alike) : Terminator
  dds_line{1..4} (4 alike) : xbsIndex_r4/DDS Compiler 6.0   partspresent=SIN_COS_LUT_only  dds_clock_rate=100  channels=1  mode_of_operation=Standard  modulus=9  parameter_entry=System_Parameters  spurious_free_dynamic_range=36.00000000  frequency_resolution=0.40000000  noise_shaping=None  phase_width=ddc_phase_width  output_width=ddc_data_width  output_selection=Sine_and_Cosine  negative_sine=off  negative_cosine=off  amplitude_mode=Full_Range  memory_type=Auto  optimization_goal=Auto  dsp48_use=Minimal  resync=off  latency_configuration=Auto  latency=1  has_phase_out=off  has_aclken=off  has_aresetn=off  explicit_period=off  period=1  data_has_tlast=Not_Required  has_tready=off  s_phase_has_tuser=Not_Required  m_data_has_tuser=Not_Required  m_phase_has_tuser=Not_Required  s_phase_tuser_width=1  output_form=Twos_Complement  s_config_sync_mode=On_Vector  phase_increment=Fixed  output_frequency1=0  output_frequency2=0  output_frequency3=0  output_frequency4=0  output_frequency5=0  output_frequency6=0  output_frequency7=0  output_frequency8=0  output_frequency9=0  output_frequency10=0  output_frequency11=0  output_frequency12=0  output_frequency13=0  output_frequency14=0  output_frequency15=0  output_frequency16=0  pinc1='0'  pinc2='0'  pinc3='0'  pinc4='0'  pinc5='0'  pinc6='0'  pinc7='0'  pinc8='0'  pinc9='0'  pinc10='0'  pinc11='0'  pinc12='0'  pinc13='0'  pinc14='0'  pinc15='0'  pinc16='0'  phase_offset=None  phase_offset_angles1=0  phase_offset_angles2=0  phase_offset_angles3=0  phase_offset_angles4=0  phase_offset_angles5=0  phase_offset_angles6=0  phase_offset_angles7=0  phase_offset_angles8=0  phase_offset_angles9=0  phase_offset_angles10=0  phase_offset_angles11=0  phase_offset_angles12=0  phase_offset_angles13=0  phase_offset_angles14=0  phase_offset_angles15=0  phase_offset_angles16=0  poff1='0'  poff2='0'  poff3='0'  poff4='0'  poff5='0'  poff6='0'  poff7='0'  poff8='0'  poff9='0'  poff10='0'  poff11='0'  poff12='0'  poff13='0'  poff14='0'  poff15='0'  poff16='0'  trim_axipin_name=on  simulation_type=hybrid_sim  simulation_model=sysgen:xddsv6_0_cmodel  data_path_portlist={ 's_axis_config_tdata_poff', 's_axis_config_tdata_chan0_poff', 's_axis_config_tdata_pinc', 's_axis_config_tdata_chan0_pinc', 's_axis_phase_tdata_resync', 's_axis_phase_tdata_chan0_resync', 's_axis_phase_tdata_poff', 's_axis_phase_tdata_chan0_poff', 's_axis_phase_tdata_pinc', 's_axis_phase_tdata_chan0_pinc', 's_axis_phase_tdata_phase_in', 'm_axis_data_tdata_sine', 'm_axis_data_tdata_chan0_sine', 'm_axis_data_tdata_cosine', 'm_axis_data_tdata_chan0_cosine', 'm_axis_phase_tdata_phase_out', 'm_axis_phase_tdata_chan0_phase_out'}  por_mode=false  gui_behaviour=Sysgen  ip_name=DDS Compiler  ip_version=6.0  dsptool_ready=true  wrapper_available=true  port_translation_map={ 'aclken' => 'en', 'aresetn' => 'rst' }  ipcore_usecache=true  ipcore_useipmodelcache=true  ipcore_xco_need_fpga_part=true  ipcore_verbose=false  block_type=dds_compiler_v6_0
  data_out_re1 : Outport
  data_out_re2 : Outport  Port=2
  data_out_re3 : Outport  Port=3
  data_out_re4 : Outport  Port=4
  data_out_im1 : Outport  Port=5
  data_out_im2 : Outport  Port=6
  data_out_im3 : Outport  Port=7
  data_out_im4 : Outport  Port=8
  wires:
  CM4/1(data_out_im) -> data_out_re4/1
  CM4/2(data_out_re) -> data_out_im4/1
  CM3/1(data_out_im) -> data_out_re3/1
  CM3/2(data_out_re) -> data_out_im3/1
  CM2/1(data_out_im) -> data_out_re2/1
  CM2/2(data_out_re) -> data_out_im2/1
  CM1/2(data_out_re) -> data_out_im1/1
  CM1/1(data_out_im) -> data_out_re1/1
  data_im4/1 -> CM4/2(data_im)
  data_im3/1 -> CM3/2(data_im)
  data_im2/1 -> CM2/2(data_im)
  data_im1/1 -> CM1/2(data_im)
  data_re4/1 -> CM4/1(data_re)
  data_re3/1 -> CM3/1(data_re)
  data_re2/1 -> CM2/1(data_re)
  data_re1/1 -> CM1/1(data_re)
  dds_line2/2 -> CM2/3(sin)
  dds_line3/2 -> CM3/3(sin)
  dds_line4/2 -> CM4/3(sin)
  dds_line4/3 -> CM4/4(cosin)
  dds_line3/3 -> CM3/4(cosin)
  dds_line2/3 -> CM2/4(cosin)
  dds_line1/2 -> CM1/3(sin)
  dds_line1/3 -> CM1/4(cosin)
  Accumulator/1 -> Register/1, AddSub/1, AddSub2/1, AddSub1/1
  phase_inc/1 -> CMult3/1, CMult1/1, CMult2/1, CMult4/1
  CMult4/1 -> AddSub1/2
  CMult2/1 -> AddSub2/2
  CMult1/1 -> AddSub/2
  dds_line4/1 -> Terminator/1
  dds_line2/1 -> Terminator2/1
  dds_line1/1 -> Terminator3/1
  dds_line3/1 -> Terminator1/1
  AddSub/1 -> dds_line2/2
  AddSub1/1 -> dds_line4/2
  AddSub2/1 -> dds_line3/2
  CMult3/1 -> Accumulator/1
  Register/1 -> dds_line1/2
  Constant/1 -> dds_line2/1, dds_line3/1, dds_line4/1, dds_line1/1
